simulink model "FAST_dissipativity_indiv"  (R2019b)
settings: Solver=ode4  StartTime=0.0  StopTime=700  FixedStep=DT  MaxStep=DT  RelTol=1e-3  EnableMultiTasking=on
values from neighbouring files (symbols this model uses):
  Alpha = exp(-2*pi*Ts*fc)    [PitchActuator_Faults_run.m]
  c = rho*A*R    [PitchActuator_Faults_run.m]
  J = 43784700    [PitchActuator_Faults_run.m]
  ki = 900    [PitchActuator_Faults_run.m]
  kp = 2000    [PitchActuator_Faults_run.m]
  m1 = 5.6    [PitchActuator_Faults_run.m]
  m2 = 0.17    [PitchActuator_Faults_run.m]
  m3 = 72.22    [PitchActuator_Faults_run.m]
  omega_0 = w0    (= 1.26710903695)    [PitchActuator_Faults_run.m]
  phi_0 = 3*Beta0^2    (= 1192.8108)    [PitchActuator_Faults_run.m]
  phi_bar = 3*Beta_max^2    (= 24300)    [PitchActuator_Faults_run.m]
  wn = 11.11    [PitchActuator_Faults_run.m]
  wn2 = 5.73    [PitchActuator_Faults_run.m]
  wn3 = 3.42    [PitchActuator_Faults_run.m]
undefined symbols (not defined in the file or in its folder): Apb, Apb1, Apb2, Bpb, Bpb1, Bpb2, GenEff, Ks1, Ks2, Ks3, OutList, R2D, sigbuilder_block, strmatch, TqInitial, VS_CtInSp, VS_MaxRat, VS_MaxTq, VS_Rgn2K, VS_RtPwr, VS_Slope15, VS_Slope25, VS_SySp, wgInitial
libraries: simulink_extras x2
settings Model: Creator=bjonkman  LastModifiedBy=samel
settings DataIOCC: LimitDataPoints=on  SaveFormat=Array  SaveOutput=off  SaveTime=off  ReturnWorkspaceOutputs=off  SignalLoggingName=sigsOut
settings OptimizationCC: ExpressionDepthLimit=2147483647  LifeSpan=inf
settings DebuggingCC: SaveWithParameterizedLinksMsg=none  UnderspecifiedInitializationDetection=Classic  MergeDetectMultiDrivingBlocksExec=none  SignalResolutionControl=TryResolveAllWithWarning  MultiTaskDSMMsg=warning  MultiTaskCondExecSysMsg=none  FcnCallInpInsideContextMsg=warning  StateNameClashWarn=warning  SFUnexpectedBacktrackingDiag=warning  SFNoUnconditionalDefaultTransitionDiag=warning  SFExecutionAtInitializationDiag=none  UnderSpecifiedDimensionMsg=warning  ArithmeticOperatorsInVariantConditions=warning
settings HardwareCC: ProdBitPerPointer=32  ProdBitPerSizeT=32  ProdBitPerPtrDiffT=32  ProdLargestAtomicFloat=None  ProdIntDivRoundTo=Undefined  ProdEndianess=Unspecified  ProdWordSize=32  ProdHWDeviceType=32-bit Generic  TargetBitPerPointer=64  TargetBitPerSizeT=64  TargetBitPerPtrDiffT=64  TargetLongLongMode=on  TargetIntDivRoundTo=Zero  TargetEndianess=LittleEndian  TargetWordSize=64  TargetHWDeviceType=MATLAB Host  ProdEqTarget=off
settings ModelReferenceCC: PropagateSignalLabelsOutOfModel=off
settings SFSimCC: SimUseLocalCustomCode=off  CustomCodeUndefinedFunction=UseInterfaceOnly
settings RTWCC: RTWUseLocalCustomCode=off
settings CodeAppCC: StateflowObjectComments=on
settings GRTTargetCC: TargetLangStandard=C89/C90 (ANSI)  GeneratePreprocessorConditionals=Disable all  CombineOutputUpdateFcns=off  GRTInterface=on
settings ConfigComp: CovMetricSettings=dw  CovHtmlReporting=on  CovSaveCumulativeToWorkspaceVar=on  CovSaveSingleToWorkspaceVar=on  CovExternalEMLEnable=off

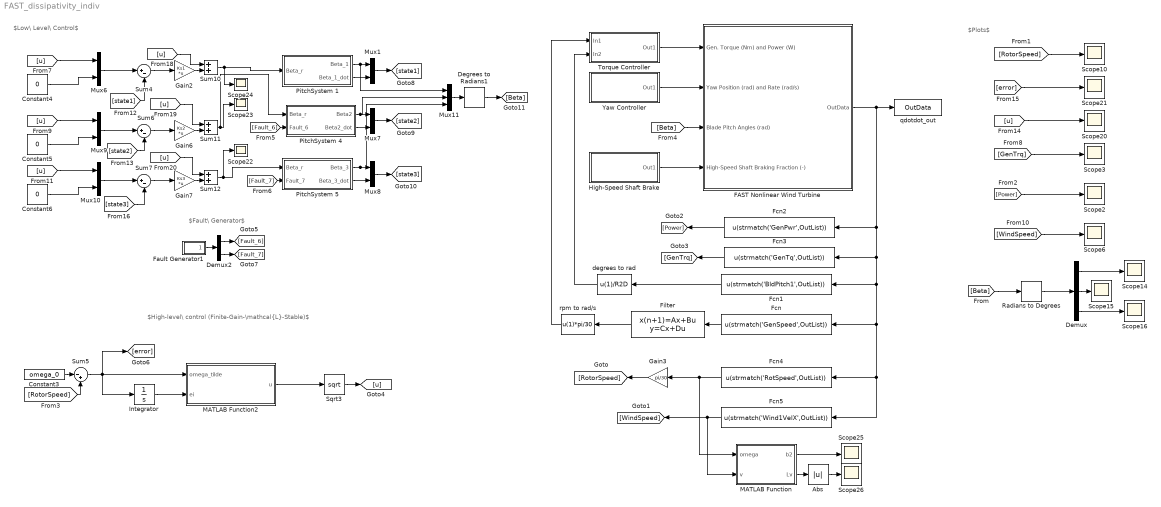
== system FAST_dissipativity_indiv ==
  note: $Plots$
  note: $Low\ Level\ Control$
  note: $Fault\ Generator$
  note: $High-level\ control (Finite-Gain-\mathcal{L}-Stable)$
  Abs : Abs
  Constant3 : Constant  Value=omega_0
  Constant4 : Constant  Value=0
  Constant5 : Constant  Value=0
  Constant6 : Constant  Value=0
  Degrees to Radians1 : simulink_extras/Transformations/Degrees to Radians
  Demux : Demux  Outputs=3
  Demux2 : Demux  Outputs=2
  FAST Nonlinear Wind Turbine : Subsystem  mask(FAST Nonlinear Wind Turbine){}
      mask help: This block contains the FAST S-Function.
      mask init:
      | clear FAST_SFunc
  Fault Generator1 : Subsystem
  Fcn : Fcn  Expr=u(strmatch('GenSpeed',OutList))
  Fcn1 : Fcn  Expr=u(strmatch('BldPitch1',OutList))
  Fcn2 : Fcn  Expr=u(strmatch('GenPwr',OutList))
  Fcn3 : Fcn  Expr=u(strmatch('GenTq',OutList))
  Fcn4 : Fcn  Expr=u(strmatch('RotSpeed',OutList))
  Fcn5 : Fcn  Expr=u(strmatch('Wind1VelX',OutList))
  Filter : DiscreteStateSpace  A=Alpha  B=1 - Alpha  C=Alpha  D=1 - Alpha  InitialCondition=wgInitial  SampleTime=-1
  Gain2 : Gain  Gain=Ks1  Multiplication=Matrix(K*u) (u vector)
  Gain3 : Gain  Gain=pi/30
  Gain6 : Gain  Gain=Ks2  Multiplication=Matrix(K*u) (u vector)
  Gain7 : Gain  Gain=Ks3  Multiplication=Matrix(K*u) (u vector)
  High-Speed Shaft Brake : Subsystem
  Integrator : Integrator
  MATLAB Function : MATLAB Function  TreatAsAtomicUnit=on
  MATLAB Function2 : MATLAB Function  TreatAsAtomicUnit=on
  Mux{1,6..10} (6 alike) : Mux  Inputs=2
  Mux11 : Mux  Inputs=3
  PitchSystem 1 : Subsystem
  PitchSystem 4 : Subsystem
  PitchSystem 5 : Subsystem
  Radians to Degrees : simulink_extras/Transformations/Radians to Degrees
  Scope{2..3,6,10,14..16,20..26} (14 alike) : Scope
  Sqrt3 : Sqrt  SaturateOnIntegerOverflow=on
  Sum10 : Sum
  Sum11 : Sum
  Sum12 : Sum
  Sum4 : Sum  Inputs=|+-
  Sum5 : Sum  Inputs=|-+
  Sum6 : Sum  Inputs=|+-
  Sum7 : Sum  Inputs=|+-
  Torque Controller : Subsystem
  Yaw Controller : Subsystem
  degrees to rad : Fcn  Expr=u(1)/R2D
  qdotdot_out : ToWorkspace  VariableName=OutData  SampleTime=-1
  rpm to rad/s : Fcn  Expr=u(1)*pi/30
  wires:
  FAST Nonlinear Wind Turbine/1(OutData) -> Fcn3/1, Fcn1/1, Fcn5/1, Fcn4/1, Fcn/1, Fcn2/1, qdotdot_out/1
  Yaw Controller/1(Out1) -> FAST Nonlinear Wind Turbine/2(Yaw Position (rad) and Rate (rad/s))
  High-Speed Shaft Brake/1(Out1) -> FAST Nonlinear Wind Turbine/4(High-Speed Shaft Braking Fraction (-))
  rpm to rad/s/1 -> Torque Controller/1(In1)
  Fcn1/1 -> degrees to rad/1
  degrees to rad/1 -> Torque Controller/2(In2)
  Fcn2/1 -> [Power]
  Fcn/1 -> Filter/1
  Filter/1 -> rpm to rad/s/1
  Fcn5/1 -> [WindSpeed], MATLAB Function/2(v)
  Fcn3/1 -> [GenTrq]
  Fcn4/1 -> MATLAB Function/1(omega), Gain3/1
  [Beta] -> FAST Nonlinear Wind Turbine/3(Blade Pitch Angles (rad))
  Torque Controller/1(Out1) -> FAST Nonlinear Wind Turbine/1(Gen. Torque (Nm) and Power (W))
  Gain3/1 -> [RotorSpeed]
  [Beta] -> Radians to Degrees/1
  Demux/1 -> Scope14/1
  Radians to Degrees/1 -> Demux/1
  Demux/2 -> Scope15/1
  Demux/3 -> Scope16/1
  Sum5/1 -> [error], Integrator/1, MATLAB Function2/1(omega_tilde)
  [RotorSpeed] -> Sum5/2
  MATLAB Function2/1(u) -> Sqrt3/1
  Constant3/1 -> Sum5/1
  Fault Generator1/1(Faults) -> Demux2/1
  [Fault_7] -> PitchSystem 5/2(Fault_7)
  Demux2/1 -> [Fault_6]
  Demux2/2 -> [Fault_7]
  [Fault_6] -> PitchSystem 4/2(Fault_6)
  Constant4/1 -> Mux6/2
  [u] -> Mux6/1
  Mux1/1 -> [state1]
  PitchSystem 1/2(Beta_1_dot) -> Mux1/2
  PitchSystem 1/1("Beta_1 ") -> Mux11/1, Mux1/1
  PitchSystem 4/1("Beta2 ") -> Mux11/2, Mux7/1
  Mux7/1 -> [state2]
  PitchSystem 4/2("Beta2_dot ") -> Mux7/2
  PitchSystem 5/1(Beta_3) -> Mux11/3, Mux8/1
  Mux8/1 -> [state3]
  PitchSystem 5/2(Beta_3_dot) -> Mux8/2
  [u] -> Mux9/1
  Constant5/1 -> Mux9/2
  Constant6/1 -> Mux10/2
  [u] -> Mux10/1
  Mux6/1 -> Sum4/1
  Mux9/1 -> Sum6/1
  Mux10/1 -> Sum7/1
  [state1] -> Sum4/2
  [state2] -> Sum6/2
  [state3] -> Sum7/2
  Gain2/1 -> Sum10/2
  Gain6/1 -> Sum11/2
  Gain7/1 -> Sum12/2
  Sum7/1 -> Gain7/1
  Sum6/1 -> Gain6/1
  Sum4/1 -> Gain2/1
  Sum10/1 -> Scope24/1, PitchSystem 1/1(Beta_r)
  Sum11/1 -> Scope23/1, PitchSystem 4/1(Beta_r)
  Sum12/1 -> Scope22/1, PitchSystem 5/1(Beta_r)
  [u] -> Sum10/1
  [u] -> Sum11/1
  [u] -> Sum12/1
  Degrees to Radians1/1 -> [Beta]
  Mux11/1 -> Degrees to Radians1/1
  Integrator/1 -> MATLAB Function2/2(ei)
  Sqrt3/1 -> [u]
  MATLAB Function/1(b2) -> Scope25/1
  MATLAB Function/2(Lv) -> Abs/1
  Abs/1 -> Scope26/1
  [RotorSpeed] -> Scope10/1
  [Power] -> Scope2/1
  [GenTrq] -> Scope3/1
  [WindSpeed] -> Scope6/1
  [u] -> Scope20/1
  [error] -> Scope21/1

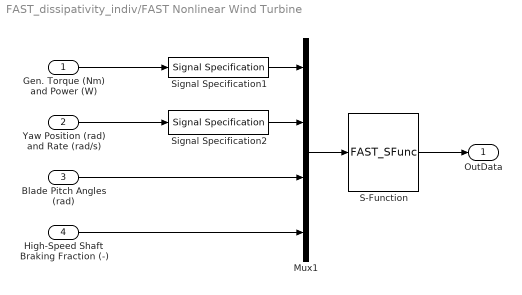
== system FAST_dissipativity_indiv/FAST Nonlinear Wind Turbine ==
  Gen. Torque (Nm) and Power (W) : Inport
  Yaw Position (rad) and Rate (rad/s) : Inport  Port=2
  Blade Pitch Angles (rad) : Inport  Port=3
  High-Speed Shaft Braking Fraction (-) : Inport  Port=4
  Mux1 : Mux
  S-Function : S-Function  FunctionName=FAST_SFunc  Parameters=FAST_InputFileName, TMax, 0  SFunctionDeploymentMode=off  EnableBusSupport=off
  Signal Specification1 : SignalSpecification  OutDataTypeStr=double  Dimensions=2
  Signal Specification2 : SignalSpecification  OutDataTypeStr=double  Dimensions=2
  OutData : Outport  VectorParamsAs1DForOutWhenUnconnected=off
  wires:
  Gen. Torque (Nm) and Power (W)/1 -> Signal Specification1/1
  S-Function/1 -> OutData/1
  Mux1/1 -> S-Function/1
  Blade Pitch Angles (rad)/1 -> Mux1/3
  Yaw Position (rad) and Rate (rad/s)/1 -> Signal Specification2/1
  Signal Specification1/1 -> Mux1/1
  Signal Specification2/1 -> Mux1/2
  High-Speed Shaft Braking Fraction (-)/1 -> Mux1/4

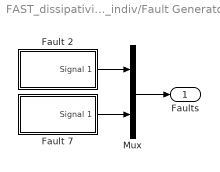
== system FAST_dissipativity_indiv/Fault Generator1 ==
  Fault 2 : Subsystem  Tag=STV Subsys  LoadFcn=sigbuilder_block('load');  StartFcn=sigbuilder_block('start');  StopFcn=sigbuilder_block('stop');  ClipboardFcn=sigbuilder_block('clipboard');  mask(Sigbuilder block){tuvar=[0:10]}
      mask help: Simulink:masks:SigbuilderBlock_MD
      mask init:
      | if ~strcmp(get_param(bdroot(gcbh),'SimulationStatus'),'stopped') tuvar = sigbuilder_block('maskInit'); end
      settings: CopyFcn=sigbuilder_block('copy');  DeleteFcn=sigbuilder_block('delete');  ModelCloseFcn=sigbuilder_block('modelClose');  PreSaveFcn=sigbuilder_block('preSave');  PauseFcn=sigbuilder_block('pause');  ContinueFcn=sigbuilder_block('continue');  NameChangeFcn=sigbuilder_block('namechange');  OpenFcn=sigbuilder_block('open',[232.8 23.4 550.8 400.2 ]);  CloseFcn=sigbuilder_block('close');
      mask Display: plot(0, 0, 100, 100,[2, 2, 32, 32, 2], [68, 8, 8, 68, 68],[32, 2], [38, 38], [32, 19, 2],[53, 60, 44], [32, 17, 17, 2],[16, 16, 31, 31]);txt = getActiveGroup(gcbh);text(2, 100, txt,'verticalAlignment', 'top');
  Fault 7 : Subsystem  Tag=STV Subsys  LoadFcn=sigbuilder_block('load');  StartFcn=sigbuilder_block('start');  StopFcn=sigbuilder_block('stop');  ClipboardFcn=sigbuilder_block('clipboard');  mask(Sigbuilder block){tuvar=[0:10]}
      mask help: Simulink:masks:SigbuilderBlock_MD
      mask init:
      | if ~strcmp(get_param(bdroot(gcbh),'SimulationStatus'),'stopped') tuvar = sigbuilder_block('maskInit'); end
      settings: CopyFcn=sigbuilder_block('copy');  DeleteFcn=sigbuilder_block('delete');  ModelCloseFcn=sigbuilder_block('modelClose');  PreSaveFcn=sigbuilder_block('preSave');  PauseFcn=sigbuilder_block('pause');  ContinueFcn=sigbuilder_block('continue');  NameChangeFcn=sigbuilder_block('namechange');  OpenFcn=sigbuilder_block('open',[437.6 199.2 550.4 400 ]);  CloseFcn=sigbuilder_block('close');
      mask Display: plot(0, 0, 100, 100,[2, 2, 32, 32, 2], [68, 8, 8, 68, 68],[32, 2], [38, 38], [32, 19, 2],[53, 60, 44], [32, 17, 17, 2],[16, 16, 31, 31]);txt = getActiveGroup(gcbh);text(2, 100, txt,'verticalAlignment', 'top');
  Mux : Mux  Inputs=2
  Faults : Outport
  wires:
  Fault 7/1(Signal 1) -> Mux/2
  Fault 2/1(Signal 1) -> Mux/1
  Mux/1 -> Faults/1

== system FAST_dissipativity_indiv/High-Speed Shaft Brake ==
  High-Speed Shaft Braking Fraction : Constant  Value=0
  Out1 : Outport  VectorParamsAs1DForOutWhenUnconnected=off
  wires:
  High-Speed Shaft Braking Fraction/1 -> Out1/1

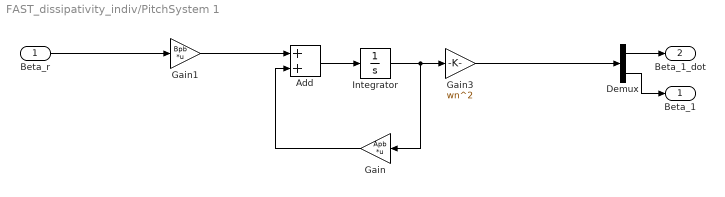
== system FAST_dissipativity_indiv/PitchSystem 1 ==
  Beta_r : Inport
  Add : Sum
  Demux : Demux  Outputs=2
  Gain : Gain  Gain=Apb  Multiplication=Matrix(K*u)
  Gain1 : Gain  Gain=Bpb  Multiplication=Matrix(K*u)
  Gain3 : Gain  Gain=wn^2
  Integrator : Integrator
  "Beta_1 " : Outport
  Beta_1_dot : Outport  Port=2
  wires:
  Gain/1 -> Add/2
  Integrator/1 -> Gain3/1, Gain/1
  Add/1 -> Integrator/1
  Gain1/1 -> Add/1
  Gain3/1 -> Demux/1
  Beta_r/1 -> Gain1/1
  Demux/1 -> Beta_1_dot/1
  Demux/2 -> "Beta_1 "/1

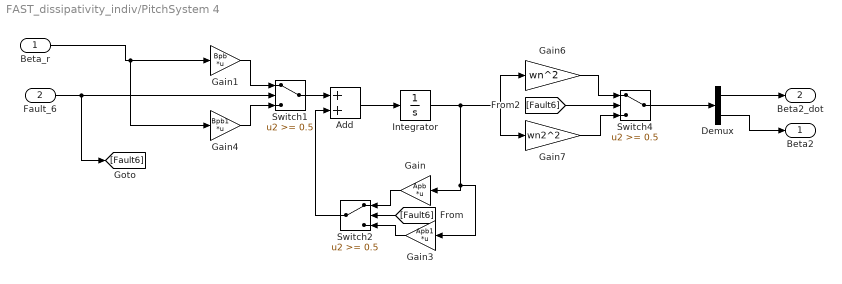
== system FAST_dissipativity_indiv/PitchSystem 4 ==
  Beta_r : Inport
  Fault_6 : Inport  Port=2
  Add : Sum
  Demux : Demux  Outputs=2
  Gain : Gain  Gain=Apb  Multiplication=Matrix(K*u)
  Gain1 : Gain  Gain=Bpb  Multiplication=Matrix(K*u)
  Gain3 : Gain  Gain=Apb1  Multiplication=Matrix(K*u)
  Gain4 : Gain  Gain=Bpb1  Multiplication=Matrix(K*u)
  Gain6 : Gain  Gain=wn^2
  Gain7 : Gain  Gain=wn2^2
  Integrator : Integrator
  Switch1 : Switch  Threshold=0.5
  Switch2 : Switch  Threshold=0.5
  Switch4 : Switch  Threshold=0.5
  "Beta2 " : Outport
  "Beta2_dot " : Outport  Port=2
  wires:
  Integrator/1 -> Gain7/1, Gain6/1, Gain/1, Gain3/1
  Add/1 -> Integrator/1
  Switch1/1 -> Add/1
  Gain1/1 -> Switch1/1
  Gain4/1 -> Switch1/3
  Gain/1 -> Switch2/1
  Gain3/1 -> Switch2/3
  Switch2/1 -> Add/2
  Fault_6/1 -> [Fault6], Switch1/2
  Beta_r/1 -> Gain1/1, Gain4/1
  [Fault6] -> Switch2/2
  [Fault6] -> Switch4/2
  Gain6/1 -> Switch4/1
  Gain7/1 -> Switch4/3
  Switch4/1 -> Demux/1
  Demux/1 -> "Beta2_dot "/1
  Demux/2 -> "Beta2 "/1

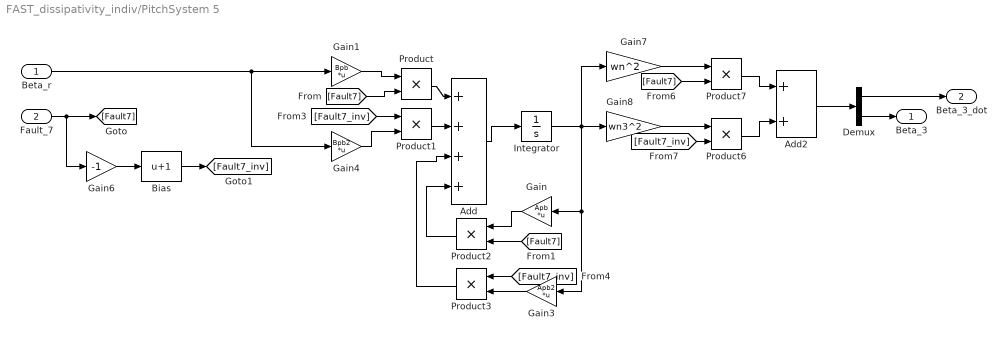
== system FAST_dissipativity_indiv/PitchSystem 5 ==
  Beta_r : Inport
  Fault_7 : Inport  Port=2
  Add : Sum  Inputs=++++
  Add2 : Sum
  Bias : Bias  Bias=1
  Demux : Demux  Outputs=2
  Gain : Gain  Gain=Apb  Multiplication=Matrix(K*u)
  Gain1 : Gain  Gain=Bpb  Multiplication=Matrix(K*u)
  Gain3 : Gain  Gain=Apb2  Multiplication=Matrix(K*u)
  Gain4 : Gain  Gain=Bpb2  Multiplication=Matrix(K*u)
  Gain6 : Gain  Gain=-1
  Gain7 : Gain  Gain=wn^2
  Gain8 : Gain  Gain=wn3^2
  Integrator : Integrator
  Product{,1..3,6..7} (6 alike) : Product  RndMeth=Zero
  Beta_3 : Outport
  Beta_3_dot : Outport  Port=2
  wires:
  Beta_r/1 -> Gain4/1, Gain1/1
  Fault_7/1 -> [Fault7], Gain6/1
  Gain4/1 -> Product1/2
  Add/1 -> Integrator/1
  Product/1 -> Add/1
  Gain1/1 -> Product/1
  Product1/1 -> Add/2
  Gain3/1 -> Product3/2
  Gain/1 -> Product2/1
  Product2/1 -> Add/4
  Product3/1 -> Add/3
  Gain6/1 -> Bias/1
  [Fault7] -> Product/2
  [Fault7] -> Product2/2
  Bias/1 -> [Fault7_inv]
  [Fault7_inv] -> Product1/1
  [Fault7_inv] -> Product3/1
  Integrator/1 -> Gain3/1, Gain/1, Gain8/1, Gain7/1
  Gain7/1 -> Product7/1
  [Fault7] -> Product7/2
  [Fault7_inv] -> Product6/2
  Gain8/1 -> Product6/1
  Product7/1 -> Add2/1
  Product6/1 -> Add2/2
  Add2/1 -> Demux/1
  Demux/2 -> Beta_3/1
  Demux/1 -> Beta_3_dot/1

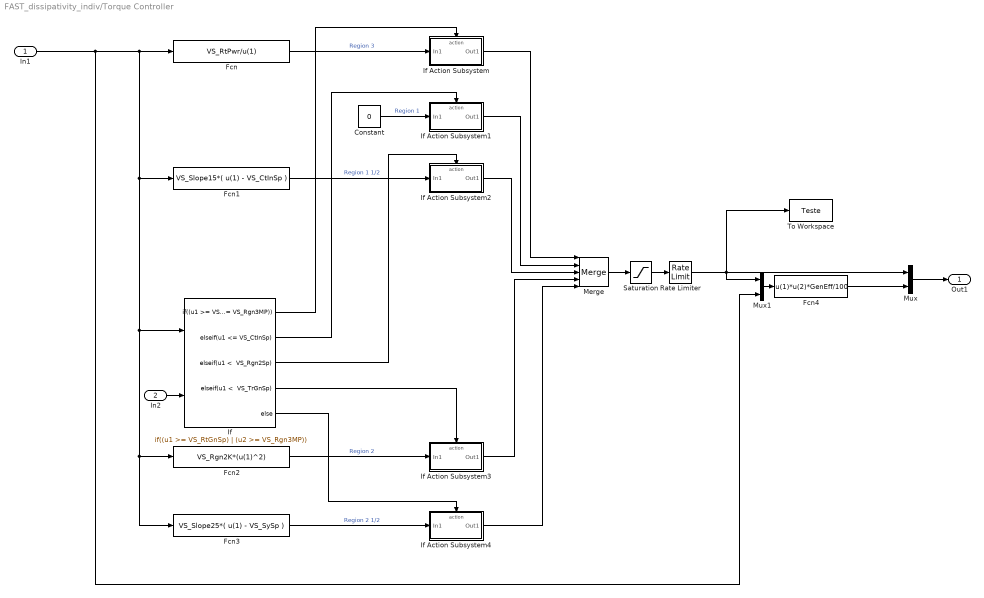
== system FAST_dissipativity_indiv/Torque Controller ==
  In1 : Inport
  In2 : Inport  Port=2
  Constant : Constant  Value=0
  Fcn : Fcn  Expr=VS_RtPwr/u(1)
  Fcn1 : Fcn  Expr=VS_Slope15*( u(1) - VS_CtInSp )
  Fcn2 : Fcn  Expr=VS_Rgn2K*(u(1)^2)
  Fcn3 : Fcn  Expr=VS_Slope25*( u(1) - VS_SySp )
  Fcn4 : Fcn  Expr=u(1)*u(2)*GenEff/100
  If : If  NumInputs=2  IfExpression=(u1 >= VS_RtGnSp) | (u2 >= VS_Rgn3MP)  ElseIfExpressions="u1 <= VS_CtInSp, u1 <  VS_Rgn2Sp, u1 <  VS_TrGnSp"
  If Action Subsystem : Subsystem  TreatAsAtomicUnit=on
  If Action Subsystem1 : Subsystem  TreatAsAtomicUnit=on
  If Action Subsystem2 : Subsystem  TreatAsAtomicUnit=on
  If Action Subsystem3 : Subsystem  TreatAsAtomicUnit=on
  If Action Subsystem4 : Subsystem  TreatAsAtomicUnit=on
  Merge : Merge  Inputs=5  InitialOutput=TqInitial
  Mux : Mux  Inputs=2
  Mux1 : Mux  Inputs=2
  Rate Limiter : RateLimiter  RisingSlewLimit=VS_MaxRat  FallingSlewLimit=-VS_MaxRat  SampleTimeMode=inherited
  Saturation : Saturate  UpperLimit=VS_MaxTq  LowerLimit=0
  To Workspace : ToWorkspace  VariableName=Teste  SaveFormat=Timeseries  SampleTime=-1
  Out1 : Outport  VectorParamsAs1DForOutWhenUnconnected=off
  wires:
  Mux/1 -> Out1/1
  Fcn/1 -> If Action Subsystem/1(In1)  "Region 3"
  If/1 -> If Action Subsystem/Action
  Constant/1 -> If Action Subsystem1/1(In1)  "Region 1"
  If/2 -> If Action Subsystem1/Action
  If/3 -> If Action Subsystem2/Action
  Fcn1/1 -> If Action Subsystem2/1(In1)  "Region 1 1/2"
  If/4 -> If Action Subsystem3/Action
  Fcn2/1 -> If Action Subsystem3/1(In1)  "Region 2"
  If/5 -> If Action Subsystem4/Action
  Fcn3/1 -> If Action Subsystem4/1(In1)  "Region 2 1/2"
  If Action Subsystem/1(Out1) -> Merge/1
  If Action Subsystem1/1(Out1) -> Merge/2
  If Action Subsystem2/1(Out1) -> Merge/3
  If Action Subsystem3/1(Out1) -> Merge/4
  If Action Subsystem4/1(Out1) -> Merge/5
  Mux1/1 -> Fcn4/1
  In1/1 -> Fcn1/1, Fcn2/1, Fcn3/1, If/1, Fcn/1, Mux1/2
  Fcn4/1 -> Mux/2
  Merge/1 -> Saturation/1
  Saturation/1 -> Rate Limiter/1
  In2/1 -> If/2
  Rate Limiter/1 -> To Workspace/1, Mux/1, Mux1/1

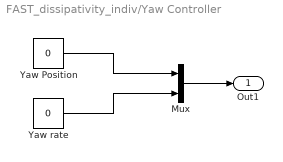
== system FAST_dissipativity_indiv/Yaw Controller ==
  Mux : Mux  Inputs=2
  Yaw Position : Constant  Value=0
  Yaw rate : Constant  Value=0
  Out1 : Outport  VectorParamsAs1DForOutWhenUnconnected=off
  wires:
  Mux/1 -> Out1/1
  Yaw Position/1 -> Mux/1
  Yaw rate/1 -> Mux/2

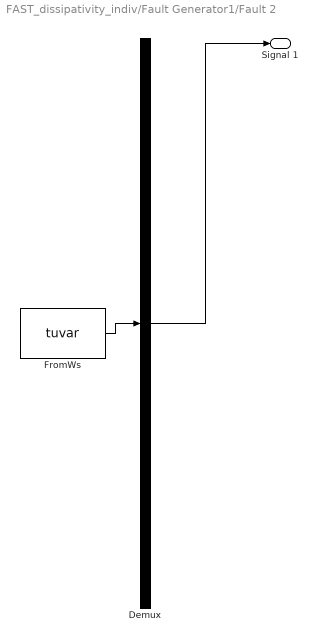
== system FAST_dissipativity_indiv/Fault Generator1/Fault 2 ==
  Demux : Demux  Tag=STV Demux  Outputs=1
  FromWs : FromWorkspace  Tag=STV FromWs  VariableName=tuvar  SampleTime=0
      SigBuilderData=|
      | common.afterFinalStr = 'Extrapolate'
      | common.sampleTime = 0
      | dataSet.timeRange = [0 600]
      | dataSet.name = 'Group 1'
      | sbobj.Groups.Name = 'Group 1'
      | sbobj.Groups.Signals.Name = 'Signal 1'
      | sbobj.Groups.Signals.XData = [0 150 150 200 200 600]
      | sbobj.Groups.Signals.YData = [1 1 0 0 1 1]
      | sbobj.Groups.TimeRange = [0 600]
  Signal 1 : Outport  Tag=STV Outport
  wires:
  Demux/1 -> Signal 1/1
  FromWs/1 -> Demux/1

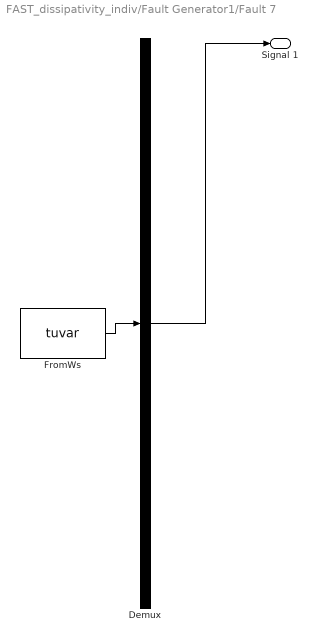
== system FAST_dissipativity_indiv/Fault Generator1/Fault 7 ==
  Demux : Demux  Tag=STV Demux  Outputs=1
  FromWs : FromWorkspace  Tag=STV FromWs  VariableName=tuvar  SampleTime=0
      SigBuilderData=|
      | common.afterFinalStr = 'Extrapolate'
      | common.sampleTime = 0
      | dataSet.timeRange = [0 800]
      | dataSet.name = 'Group 1'
      | sbobj.Groups.Name = 'Group 1'
      | sbobj.Groups.Signals.Name = 'Signal 1'
      | sbobj.Groups.Signals.XData = [0 250 280 320 350 800]
      | sbobj.Groups.Signals.YData = [1 1 0 0 1 1]
      | sbobj.Groups.TimeRange = [0 800]
  Signal 1 : Outport  Tag=STV Outport
  wires:
  Demux/1 -> Signal 1/1
  FromWs/1 -> Demux/1

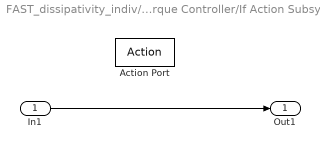
== system FAST_dissipativity_indiv/Torque Controller/If Action Subsystem ==
  In1 : Inport
  Action Port : ActionPort  ActionPortLabel=if((u1 >= VS_RtGnSp) | (u2 >= VS_Rgn3MP))
  Out1 : Outport  VectorParamsAs1DForOutWhenUnconnected=off
  wires:
  In1/1 -> Out1/1

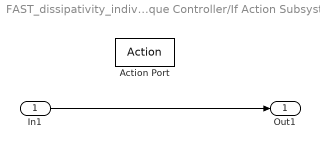
== system FAST_dissipativity_indiv/Torque Controller/If Action Subsystem1 ==
  In1 : Inport
  Action Port : ActionPort  ActionPortLabel=elseif(u1 <= VS_CtInSp)
  Out1 : Outport  VectorParamsAs1DForOutWhenUnconnected=off
  wires:
  In1/1 -> Out1/1

== system FAST_dissipativity_indiv/Torque Controller/If Action Subsystem2 ==
  In1 : Inport
  Action Port : ActionPort  ActionPortLabel="elseif( u1 <  VS_Rgn2Sp)"
  Out1 : Outport  VectorParamsAs1DForOutWhenUnconnected=off
  wires:
  In1/1 -> Out1/1

== system FAST_dissipativity_indiv/Torque Controller/If Action Subsystem3 ==
  In1 : Inport
  Action Port : ActionPort  ActionPortLabel="elseif( u1 <  VS_TrGnSp)"
  Out1 : Outport  VectorParamsAs1DForOutWhenUnconnected=off
  wires:
  In1/1 -> Out1/1

== system FAST_dissipativity_indiv/Torque Controller/If Action Subsystem4 ==
  In1 : Inport
  Action Port : ActionPort  ActionPortLabel=else
  Out1 : Outport  VectorParamsAs1DForOutWhenUnconnected=off
  wires:
  In1/1 -> Out1/1

== matlab function FAST_dissipativity_indiv/MATLAB Function2 ==
  data: omega_tilde input; u output; phi_0 parameter; phi_bar parameter; ei input; kp parameter; ki parameter
function u = fcn(omega_tilde,phi_0,phi_bar,ei,kp,ki)
x1=-phi_0;
x2=phi_bar-phi_0;
u=phi_0+sat(kp*omega_tilde+ki*ei,x1,x2);

== matlab function FAST_dissipativity_indiv/MATLAB Function ==
  data: b2 output; omega input; v input; Lv output; m1 parameter; m2 parameter; m3 parameter; J parameter; c parameter
function [b2,Lv] = fcn(omega,v, m1, m2, m3, J,c)
e      =    exp(-m2*v/omega);
b2     =    (c*v^3/(6*J*omega))*m3*e;
Lv     =    ((4*c*v^3/(2*J*omega^2))-(3*m1*c*v^2/(2*J*omega)))*e-(m2/omega)*((c*v^4/(2*J*omega^2))-m1*c*v^3/(2*J*omega))*e-3*c*v^2/(6*J*omega)*m3*e+(m2/omega)*c*v^3/(6*J*omega)*m3*e;
